simulink model "PV_BoostControlTuning_ST"  (R2018b)
settings: Solver=ode23tb  StartTime=0.0  StopTime=10  MaxStep=1e-4  RelTol=1e-3
PreLoadFcn:
  | load('EmulatedPV_LowPowerData.mat');
  | 
  | numIrr = 10;
  | ArrayPower = ArrayCurrent.*ArrayVoltage;
InitFcn:
  | Ts = 1e-4;
  | Tc = Ts;
undefined symbols (not defined in the file): ArrayCurrent, ArrayVoltage, DiscIntNeverNeededParam, Irradiance
libraries: powerlib x11, simulink x1, powerlib_meascontrol x1
settings Model: Creator=jlesage  LastModifiedBy=jlesage
settings DebuggingCC: LibraryContextMissingDiagnostic=none
settings SFSimCC: SimUseLocalCustomCode=off
settings RTWCC: RTWUseLocalCustomCode=off

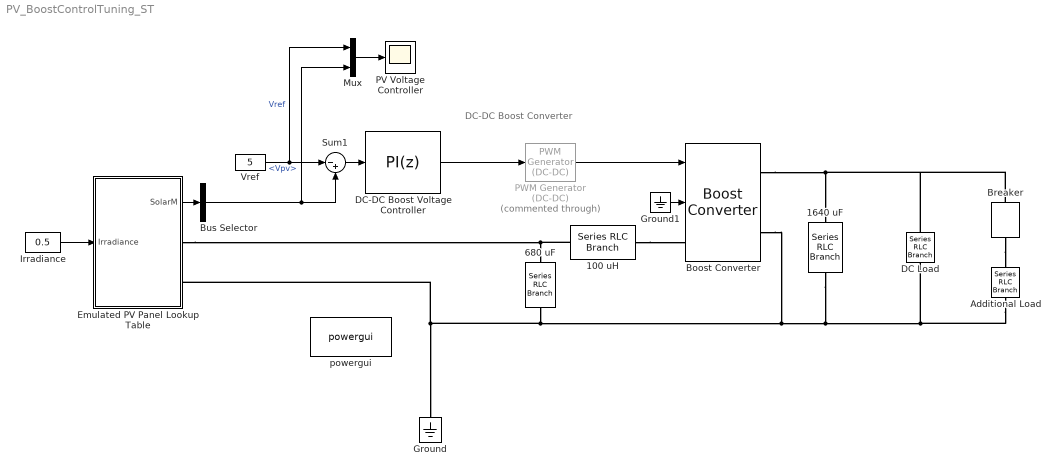
== system PV_BoostControlTuning_ST ==
  note: DC-DC Boost Converter
  100 uH : powerlib/Elements/Series RLC Branch  LConnTagsString=__new0  RConnTagsString=__new0  BranchType=L  Resistance=1  Inductance=100e-6  SetiL0=off  InitialCurrent=0  Capacitance=1e-6  Setx0=off  InitialVoltage=0  Measurements=None
      settings: SourceProductName=Simscape Electrical
  1640 uF : powerlib/Elements/Series RLC Branch  LConnTagsString=__new0  RConnTagsString=__new0  BranchType=C  Resistance=1  Inductance=1e-3  SetiL0=off  InitialCurrent=0  Capacitance=1640e-6  Setx0=on  InitialVoltage=11.2  Measurements=None
      settings: SourceProductName=Simscape Electrical
  680 uF : powerlib/Elements/Series RLC Branch  LConnTagsString=__new0  RConnTagsString=__new0  BranchType=C  Resistance=1e-3  Inductance=1e-3  SetiL0=off  InitialCurrent=0  Capacitance=680e-6  Setx0=on  InitialVoltage=5  Measurements=None
      settings: SourceProductName=Simscape Electrical
  Additional Load : powerlib/Elements/Series RLC Branch  LConnTagsString=__new0  RConnTagsString=__new0  BranchType=R  Resistance=11.5  Inductance=1e-3  SetiL0=off  InitialCurrent=0  Capacitance=1e-6  Setx0=off  InitialVoltage=0  Measurements=None
      settings: SourceProductName=Simscape Electrical
  "Boost Converter " : powerlib/Power Electronics/Boost Converter  ModelType=Average model (D-controlled)  Ron=1e-3  Rs=1e6  Cs=inf  Vforward=[0,0.8]  Ron_Diode=1e-3  Rs_Diode=1e6  Cs_Diode=inf  Vf_Diode=0.8  Rs_CurrentSource=inf
      settings: SourceProductName=Simscape Electrical  SourceProductBaseCode=PS
  Breaker : powerlib/Elements/Breaker  InitialState=0  SwitchingTimes=1  External=off  BreakerResistance=0.01  SnubberResistance=1e6  SnubberCapacitance=inf  Measurements=None  MoreParameters=on  NoBreakLoop=off
      settings: SourceProductName=Simscape Electrical
  Bus Selector : BusSelector  OutputSignals=Vpv
  DC Load : powerlib/Elements/Series RLC Branch  LConnTagsString=__new0  RConnTagsString=__new0  BranchType=R  Resistance=11.5  Inductance=1e-3  SetiL0=off  InitialCurrent=0  Capacitance=1e-6  Setx0=off  InitialVoltage=0  Measurements=None
      settings: SourceProductName=Simscape Electrical
  DC-DC Boost Voltage Controller : simulink/Continuous/PID Controller  Controller=PI  Form=Parallel  TimeDomain=Discrete-time  SampleTime=Tc  IntegratorMethod=Forward Euler  FilterMethod=Forward Euler  ControllerParametersSource=internal  P=0.1  I=0.1  D=0  UseFilter=on  N=100  TunerSelectOption=Transfer Function Based (PID Tuner App)  InitialConditionSource=internal  InitialConditionForIntegrator=0.625  InitialConditionForFilter=0  DifferentiatorICPrevScaledInput=0  ExternalReset=none  TrackingMode=off  Kt=1  LimitOutput=off  UpperSaturationLimit=0.9  LowerSaturationLimit=0  LinearizeAsGain=on  AntiWindupMode=clamping  Kb=1  POutMin=[]  POutMax=[]  IOutMin=[]  IOutMax=[]  DOutMin=[]  DOutMax=[]  NOutMin=[]  NOutMax=[]  SumOutMin=[]  SumOutMax=[]  SaturationOutMin=[]  SaturationOutMax=[]  PParamMin=[]  PParamMax=[]  IParamMin=[]  IParamMax=[]  DParamMin=[]  DParamMax=[]  NParamMin=[]  NParamMax=[]  KbParamMin=[]  KbParamMax=[]  KtParamMin=[]  KtParamMax=[]  KbOutMin=[]  KbOutMax=[]  KtOutMin=[]  KtOutMax=[]  IntegratorOutMin=[]  IntegratorOutMax=[]  FilterOutMin=[]  FilterOutMax=[]  SumI1OutMin=[]  SumI1OutMax=[]  SumI2OutMin=[]  SumI2OutMax=[]  SumI3OutMin=[]  SumI3OutMax=[]  SumI4OutMin=[]  SumI4OutMax=[]  SumDOutMin=[]  SumDOutMax=[]  DifferentiatorOutMin=[]  DifferentiatorOutMax=[]  FilterDiffOutCoefMin=[]  FilterDiffOutCoefMax=[]  ReciprocalOutMin=[]  ReciprocalOutMax=[]  SumDenOutMin=[]  SumDenOutMax=[]  SumNumOutMin=[]  SumNumOutMax=[]  DivideOutMin=[]  DivideOutMax=[]  IntegratorContinuousStateAttributes=''  IntegratorStateMustResolveToSignalObject=off  IntegratorRTWStateStorageClass=Auto  FilterContinuousStateAttributes=''  FilterStateMustResolveToSignalObject=off  FilterRTWStateStorageClass=Auto  ParallelPVariant=InternalParameters  IdealPVariant=Disabled  IVariant=InternalParameters  DVariant=Disabled  IntegratorVariant=Discrete  SatVariant=Disabled  AWVariant=Passthrough  PCopyVariant=Disabled  TRVariant=Disabled  FdbkBlocksVariant=Forward  IdealPFdbkVariant=Disabled  SatFdbkVariant=Disabled  DerivativeFilterVariant=Disabled  NVariant=Disabled  NCopyVariant=Disabled_SignalSpec  FilterICVariant=Disabled  IntegratorICVariant=InternalICs  ExternalResetVariant=Disabled  TRSumVariant=Passthrough  SumFdbkVariant=Disabled  SumVariant=Sum_PI
  Emulated PV Panel Lookup Table : Subsystem
      mask Display:
      | image(imread('panel.jpg'))
      | color('yellow')
      | port_label('input',1,'Ir')
      | port_label('output',1,'m')
      | port_label('Rconn',1,'A')
      | port_label('Rconn',2,'B')
  Ground : powerlib/Elements/Ground  LConnTagsString=a
      settings: SourceProductName=Simscape Electrical
  Ground1 : Ground
  Irradiance : Constant  Value=0.5  OutDataTypeStr=double
  Mux : Mux  Inputs=2
  PV Voltage Controller : Scope
  PWM Generator (DC-DC) : powerlib_meascontrol/Pulse & Signal Generators/PWM Generator (DC-DC)  Commented=through  Fsw=5000  Ts=Tc
      settings: SourceProductName=Simscape Electrical
  Sum1 : Sum  Inputs=|-+
  Vref : Constant  Value=5
  powergui : powerlib/powergui  Priority=1  SimulationMode=Discrete  SampleTime=Ts  frequency=60  Iterations=50  frequencyindice=0  Pbase=100e6  ErrMax=1e-4  UnitsV=kV  UnitsW=MW  buscounter=0  FunctionMessages=off  echomessages=off  EnableUseOfTLC=off  CurrentSourceSwitches=off  DisableSnubberDevices=off  DisableRonSwitches=off  DisableVfSwitches=off  DisplayEquations=off  SolverType=Tustin/Backward Euler (TBE)  Interpol=off  ExternalGateDelay=off  methode=off  Ts=100  x0status=blocks  SPID=on  SwTol=0  HookPort=off  RestoreLinks=warning  ResistiveCurrentMeasurement=off  Frange=[0:2:500]  Ylog=off  Xlog=on  ShowGrid=off  save=off  variable=ZData  structure=0  ZoomFFT=off  StartTime=0.0  cycles=1  DisplayStyle=1  fundamental=60  FreqAxis=off  MaxFrequency=1000  frequencyindicesteady=1  RmsSteady=1  display=off
  wires:
  Irradiance/1 -> Emulated PV Panel Lookup Table/1(Irradiance)
  Emulated PV Panel Lookup Table/1(SolarM) -> Bus Selector/1
  Ground1/1 -> "Boost Converter "/2
  DC-DC Boost Voltage Controller/1 -> PWM Generator (DC-DC)/1
  Sum1/1 -> DC-DC Boost Voltage Controller/1
  Bus Selector/1 -> Mux/2, Sum1/2  "<Vpv>"
  Vref/1 -> Mux/1, Sum1/1  "Vref"
  Mux/1 -> PV Voltage Controller/1
  PWM Generator (DC-DC)/1 -> "Boost Converter "/1
  connections:
  "Boost Converter "/RConn1 -- Breaker/LConn1 -- DC Load/LConn1 -- 1640 uF/LConn1
  100 uH/RConn1 -- "Boost Converter "/LConn1
  680 uF/RConn1 -- Ground/LConn1 -- Emulated PV Panel Lookup Table/RConn2 -- Additional Load/RConn1 -- DC Load/RConn1 -- 1640 uF/RConn1 -- "Boost Converter "/RConn2
  100 uH/LConn1 -- Emulated PV Panel Lookup Table/RConn1 -- 680 uF/LConn1
  Breaker/RConn1 -- Additional Load/LConn1

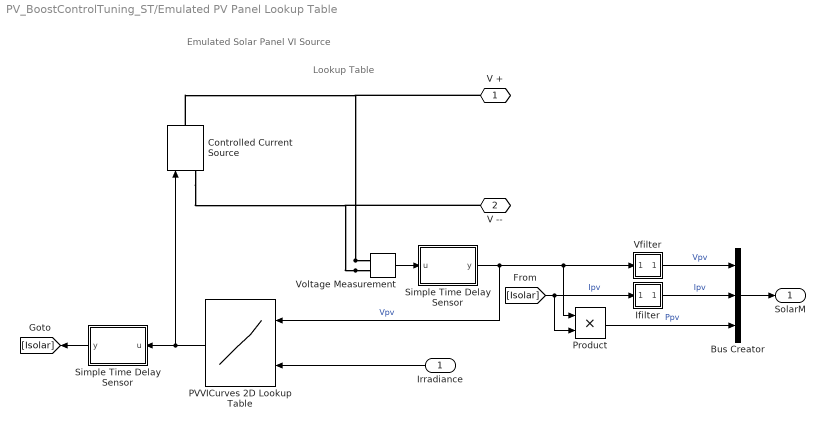
== system PV_BoostControlTuning_ST/Emulated PV Panel Lookup Table ==
  note: Lookup Table
  note: Emulated Solar Panel VI Source
  Irradiance : Inport
  Bus Creator : BusCreator  Inputs=3
  Controlled Current Source : powerlib/Electrical Sources/Controlled Current Source  Initialize=on  Source_Type=AC  Amplitude=0  Phase=0  Frequency=0  Measurements=None
      settings: SourceProductName=Simscape Electrical
  Ifilter : Subsystem  mask{Tf=0.01}
      mask prompts: Tf "Filter Time Constant"
  PVVICurves 2D Lookup Table : Lookup_n-D  BreakpointsForDimension1=ArrayVoltage  BreakpointsForDimension2=Irradiance  Table=ArrayCurrent  InternalRulePriority=Speed  RndMeth=Simplest  InputSameDT=on
  Product : Product
  Simple Time Delay Sensor : Subsystem  mask{Ts=Ts, Tau=0.0001}
      mask prompts: Ts "Sample Time, [s]"; Tau "Time Constant, Tau [s]"
      mask help: Simple Sensor
      mask Display: fprintf('1\n------------\n(1 + s Tau)');
  "Simple Time Delay Sensor " : Subsystem  mask{Ts=Ts, Tau=0.0001}
      mask prompts: Ts "Sample Time, [s]"; Tau "Time Constant, Tau [s]"
      mask help: Simple Sensor
      mask Display: fprintf('1\n------------\n(1 + s Tau)');
  Vfilter : Subsystem  mask{Tf=0.01}
      mask prompts: Tf "Filter Time Constant"
  Voltage Measurement : powerlib/Measurements/Voltage Measurement  PhasorSimulation=off  OutputType=Complex  PSBequivalent=0
      settings: SourceProductName=Simscape Electrical
  V + : PMIOPort  Side=Right
  V -- : PMIOPort  Port=2  Side=Right
  SolarM : Outport
  wires:
  Irradiance/1 -> PVVICurves 2D Lookup Table/2
  PVVICurves 2D Lookup Table/1 -> Simple Time Delay Sensor/1(u), Controlled Current Source/1
  Bus Creator/1 -> SolarM/1
  [Isolar] -> Product/2, Ifilter/1(u)  "Ipv"
  Product/1 -> Bus Creator/3  "Ppv"
  Simple Time Delay Sensor/1(y) -> [Isolar]
  "Simple Time Delay Sensor "/1(y) -> Product/1, Vfilter/1(u), PVVICurves 2D Lookup Table/1  "Vpv"
  Voltage Measurement/1 -> "Simple Time Delay Sensor "/1(u)
  Vfilter/1(y) -> Bus Creator/1  "Vpv"
  Ifilter/1(y) -> Bus Creator/2  "Ipv"
  connections:
  Voltage Measurement/LConn2 -- Controlled Current Source/LConn1 -- V --/RConn1
  Voltage Measurement/LConn1 -- Controlled Current Source/RConn1 -- V +/RConn1

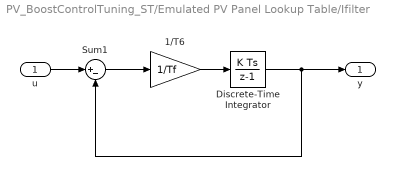
== system PV_BoostControlTuning_ST/Emulated PV Panel Lookup Table/Ifilter ==
  u : Inport
  1/T6 : Gain  Gain=1/Tf
  Discrete-Time Integrator : DiscreteIntegrator  InitialCondition=2.595  SampleTime=Tc  ICPrevOutput=DiscIntNeverNeededParam  ICPrevScaledInput=DiscIntNeverNeededParam
  Sum1 : Sum  Inputs=|+-
  y : Outport
  wires:
  Sum1/1 -> 1/T6/1
  Discrete-Time Integrator/1 -> Sum1/2, y/1
  u/1 -> Sum1/1
  1/T6/1 -> Discrete-Time Integrator/1

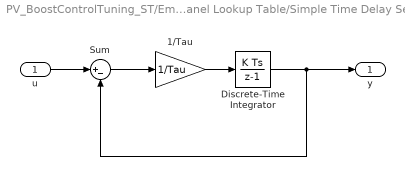
== system PV_BoostControlTuning_ST/Emulated PV Panel Lookup Table/Simple Time Delay Sensor ==
  u : Inport
  1/Tau : Gain  Gain=1/Tau
  Discrete-Time Integrator : DiscreteIntegrator  InitialCondition=2.595  SampleTime=Ts  ICPrevOutput=DiscIntNeverNeededParam  ICPrevScaledInput=DiscIntNeverNeededParam
  Sum : Sum  Inputs=|+-
  y : Outport
  wires:
  1/Tau/1 -> Discrete-Time Integrator/1
  Sum/1 -> 1/Tau/1
  u/1 -> Sum/1
  Discrete-Time Integrator/1 -> y/1, Sum/2

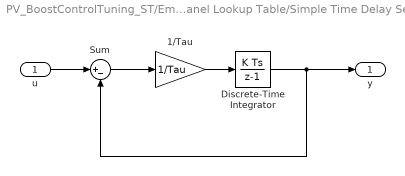
== system PV_BoostControlTuning_ST/Emulated PV Panel Lookup Table/Simple Time Delay Sensor  ==
  u : Inport
  1/Tau : Gain  Gain=1/Tau
  Discrete-Time Integrator : DiscreteIntegrator  InitialCondition=5  SampleTime=Ts  ICPrevOutput=DiscIntNeverNeededParam  ICPrevScaledInput=DiscIntNeverNeededParam
  Sum : Sum  Inputs=|+-
  y : Outport
  wires:
  Discrete-Time Integrator/1 -> Sum/2, y/1
  u/1 -> Sum/1
  Sum/1 -> 1/Tau/1
  1/Tau/1 -> Discrete-Time Integrator/1

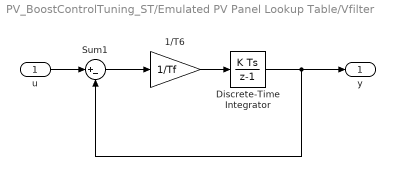
== system PV_BoostControlTuning_ST/Emulated PV Panel Lookup Table/Vfilter ==
  u : Inport
  1/T6 : Gain  Gain=1/Tf
  Discrete-Time Integrator : DiscreteIntegrator  InitialCondition=5  SampleTime=Tc  ICPrevOutput=DiscIntNeverNeededParam  ICPrevScaledInput=DiscIntNeverNeededParam
  Sum1 : Sum  Inputs=|+-
  y : Outport
  wires:
  1/T6/1 -> Discrete-Time Integrator/1
  u/1 -> Sum1/1
  Discrete-Time Integrator/1 -> y/1, Sum1/2
  Sum1/1 -> 1/T6/1
